simulink model "Pedirtiempo_Harness5"  (R2020b)
settings: Solver=VariableStepAuto  StartTime=0.0  StopTime=10.0  RelTol=1e-3
settings Model: Creator=cacha  LastModifiedBy=cacha

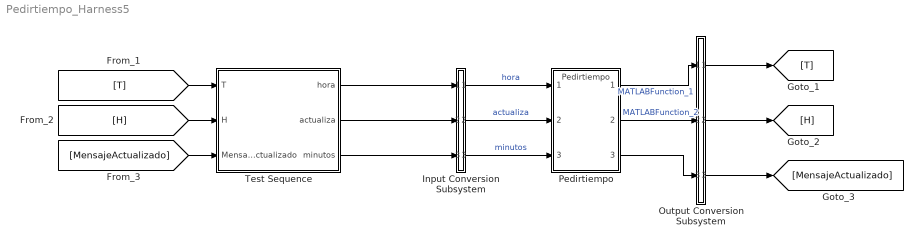
== system Pedirtiempo_Harness5 ==
  Input Conversion Subsystem : Subsystem  Tag=__SLT_ICS__  Description=|
      | Signal spec.
      | and routing
      settings: AttributesFormatString=%<Description>
  Output Conversion Subsystem : Subsystem  Tag=__SLT_OCS__  Description=|
      | Signal spec.
      | and routing
      settings: AttributesFormatString=%<Description>
  Pedirtiempo : ModelReference  ModelNameDialog=Pedirtiempo  SimulationMode=Normal  ModelReferenceVersion=1.30
  Test Sequence : Test Sequence  TreatAsAtomicUnit=on
  wires:
  Test Sequence/1(hora) -> Input Conversion Subsystem/1(Inport_1)
  Test Sequence/2(actualiza) -> Input Conversion Subsystem/2(Inport_2)
  Test Sequence/3(minutos) -> Input Conversion Subsystem/3(Inport_3)
  [T] -> Test Sequence/1(T)
  [H] -> Test Sequence/2(H)
  [MensajeActualizado] -> Test Sequence/3(MensajeActualizado)
  Output Conversion Subsystem/1(Outport_1) -> [T]
  Output Conversion Subsystem/2(Outport_2) -> [H]
  Output Conversion Subsystem/3(Outport_3) -> [MensajeActualizado]
  Input Conversion Subsystem/1(Outport_1) -> Pedirtiempo/1  "hora"
  Input Conversion Subsystem/2(Outport_2) -> Pedirtiempo/2  "actualiza"
  Input Conversion Subsystem/3(Outport_3) -> Pedirtiempo/3  "minutos"
  Pedirtiempo/1 -> Output Conversion Subsystem/1(Inport_1)  "MATLABFunction_1"
  Pedirtiempo/2 -> Output Conversion Subsystem/2(Inport_2)  "MATLABFunction_2"
  Pedirtiempo/3 -> Output Conversion Subsystem/3(Inport_3)

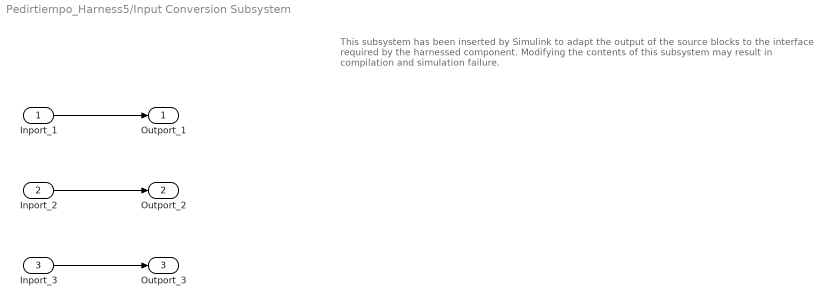
== system Pedirtiempo_Harness5/Input Conversion Subsystem ==
  note: This subsystem has been inserted by Simulink to adapt the output of the source blocks to the interface required by the harnessed component.
      |  Modifying the contents of this subsystem may result in compilation and simulation failure.
  Inport_1 : Inport
  Inport_2 : Inport  Port=2
  Inport_3 : Inport  Port=3
  Outport_1 : Outport
  Outport_2 : Outport  Port=2
  Outport_3 : Outport  Port=3
  wires:
  Inport_1/1 -> Outport_1/1
  Inport_2/1 -> Outport_2/1
  Inport_3/1 -> Outport_3/1

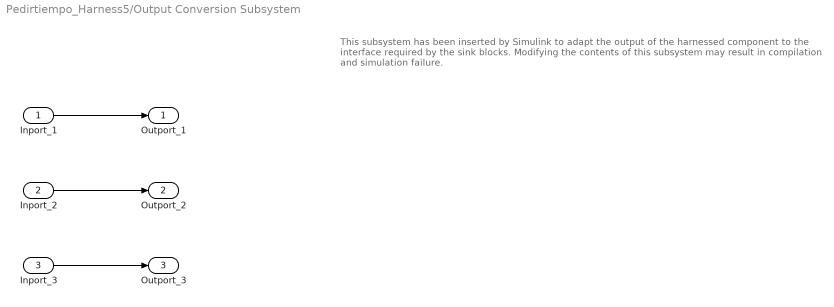
== system Pedirtiempo_Harness5/Output Conversion Subsystem ==
  note: This subsystem has been inserted by Simulink to adapt the output of the harnessed component to the interface required by the sink blocks.
      |  Modifying the contents of this subsystem may result in compilation and simulation failure.
  Inport_1 : Inport
  Inport_2 : Inport  Port=2
  Inport_3 : Inport  Port=3
  Outport_1 : Outport
  Outport_2 : Outport  Port=2
  Outport_3 : Outport  Port=3
  wires:
  Inport_1/1 -> Outport_1/1
  Inport_2/1 -> Outport_2/1
  Inport_3/1 -> Outport_3/1

== stateflow chart Pedirtiempo_Harness5/Test Sequence ==
  settings: stateMachineType=SIMPLIFIED_MACHINE
  state Run
    %% Initialize data outputs.
    hora = 0;
    actualiza = 0;
    minutos = 0;
  (default) -> Run
  data: T input double size=[1]; H input double size=[1]; MensajeActualizado input double size=[1]; hora output double size=[1]; actualiza output double size=[1]; minutos output double size=[1]
